simulink model "simIdeal"  (R2023b)
settings: Solver=VariableStepAuto  StartTime=0.0  StopTime=tf  MaxStep=1e-5  RelTol=1e-3
undefined symbols (not defined in the file): ke, p, stepTime, tPWM, Vmax, voltage
libraries: simulink x2
settings Model: Creator=miqui  LastModifiedBy=miqui

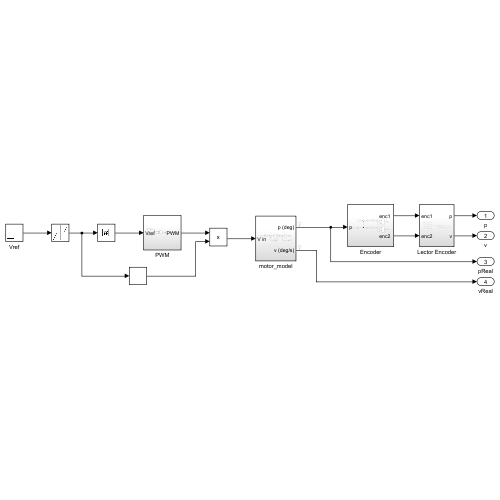
[thumbnail: Simulink's stored preview of the top-level diagram]
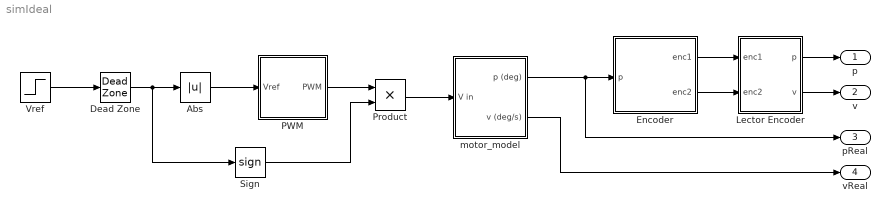
== system simIdeal ==
  Abs : Abs  SaturateOnIntegerOverflow=off
  Dead Zone : DeadZone
  Encoder : Subsystem
  Lector Encoder : Subsystem
  PWM : Subsystem
  Product : Product
  Sign : Signum
  Vref : Step  Time=stepTime  After=voltage  SampleTime=0
  motor_model : Subsystem
  p : Outport
  v : Outport  Port=2
  pReal : Outport  Port=3
  vReal : Outport  Port=4
  wires:
  Dead Zone/1 -> Sign/1, Abs/1
  Abs/1 -> PWM/1(Vref)
  PWM/1(PWM) -> Product/1
  Product/1 -> motor_model/1(V in)
  Sign/1 -> Product/2
  Vref/1 -> Dead Zone/1
  Lector Encoder/2(v) -> v/1
  Lector Encoder/1(p) -> p/1
  motor_model/2(v (deg/s)) -> vReal/1
  motor_model/1(p (deg)) -> Encoder/1(p), pReal/1
  Encoder/1("enc1 ") -> Lector Encoder/1(enc1)
  Encoder/2("enc2 ") -> Lector Encoder/2(enc2)

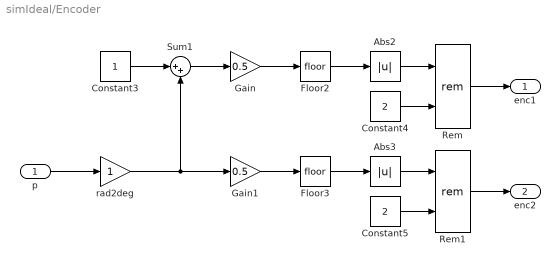
== system simIdeal/Encoder ==
  p : Inport
  Abs2 : Abs  SaturateOnIntegerOverflow=off
  Abs3 : Abs  SaturateOnIntegerOverflow=off
  Constant3 : Constant
  Constant4 : Constant  Value=2
  Constant5 : Constant  Value=2
  Floor2 : Rounding
  Floor3 : Rounding
  Gain : Gain  Gain=0.5
  Gain1 : Gain  Gain=0.5
  Rem : Math  Operator=rem
  Rem1 : Math  Operator=rem
  Sum1 : Sum  Inputs=|++
  rad2deg : Gain
  "enc1 " : Outport  SampleTime=0.0001
  "enc2 " : Outport  Port=2  SampleTime=0.0001
  wires:
  Constant4/1 -> Rem/2
  Constant3/1 -> Sum1/1
  p/1 -> rad2deg/1
  Rem1/1 -> "enc2 "/1
  Gain/1 -> Floor2/1
  Abs3/1 -> Rem1/1
  rad2deg/1 -> Gain1/1, Sum1/2
  Sum1/1 -> Gain/1
  Gain1/1 -> Floor3/1
  Floor3/1 -> Abs3/1
  Floor2/1 -> Abs2/1
  Constant5/1 -> Rem1/2
  Rem/1 -> "enc1 "/1
  Abs2/1 -> Rem/1

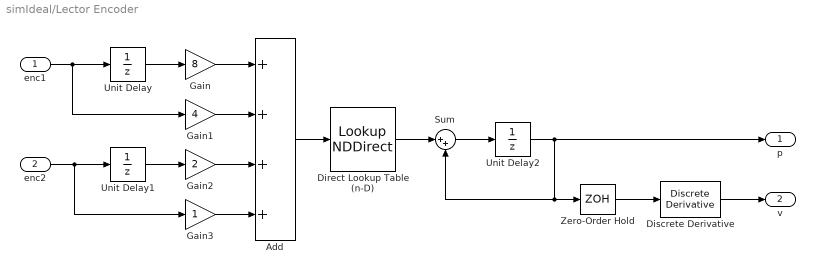
== system simIdeal/Lector Encoder ==
  enc1 : Inport
  enc2 : Inport  Port=2
  Add : Sum  Inputs=++++  OutDataTypeStr=double
  Direct Lookup Table (n-D) : LookupNDDirect  NumberOfTableDimensions=1  Table=[0,-1,1,0,1,0,0,-1,-1,0,0,1,0,1,-1,0]
  Discrete Derivative : simulink/Discrete/Discrete Derivative  gainval=1.0  ICPrevScaledInput=0.0  OutMin=[]  OutMax=[]  OutDataType=fixdt(1, 16)  OutScaling=2^-10  DoSatur=off
  Gain : Gain  Gain=8
  Gain1 : Gain  Gain=4
  Gain2 : Gain  Gain=2
  Gain3 : Gain
  Sum : Sum  Inputs=|++
  Unit Delay : UnitDelay  SampleTime=-1  HasFrameUpgradeWarning=on
  Unit Delay1 : UnitDelay  SampleTime=-1  HasFrameUpgradeWarning=on
  Unit Delay2 : UnitDelay  SampleTime=-1  HasFrameUpgradeWarning=on
  Zero-Order Hold : ZeroOrderHold  SampleTime=0.01
  p : Outport
  v : Outport  Port=2
  wires:
  enc1/1 -> Unit Delay/1, Gain1/1
  enc2/1 -> Unit Delay1/1, Gain3/1
  Unit Delay/1 -> Gain/1
  Unit Delay1/1 -> Gain2/1
  Gain/1 -> Add/1
  Gain1/1 -> Add/2
  Gain2/1 -> Add/3
  Gain3/1 -> Add/4
  Add/1 -> Direct Lookup Table (n-D)/1
  Direct Lookup Table (n-D)/1 -> Sum/1
  Sum/1 -> Unit Delay2/1
  Unit Delay2/1 -> Zero-Order Hold/1, Sum/2, p/1
  Zero-Order Hold/1 -> Discrete Derivative/1
  Discrete Derivative/1 -> v/1

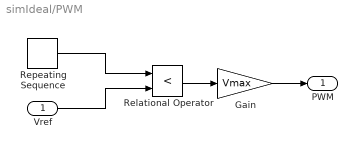
== system simIdeal/PWM ==
  Vref : Inport
  Gain : Gain  Gain=Vmax
  Relational Operator : RelationalOperator  Operator=<  OutDataTypeStr=boolean  RndMeth=Simplest  InputSameDT=off
  Repeating Sequence : simulink/Sources/Repeating Sequence  rep_seq_t=linspace(0,tPWM,100)  rep_seq_y=linspace(0,Vmax,100)
  PWM : Outport
  wires:
  Relational Operator/1 -> Gain/1
  Gain/1 -> PWM/1
  Vref/1 -> Relational Operator/2
  Repeating Sequence/1 -> Relational Operator/1

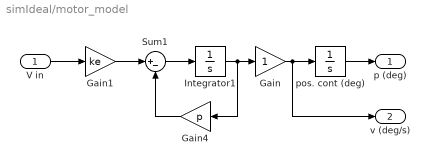
== system simIdeal/motor_model ==
  V in : Inport
  Gain : Gain
  Gain1 : Gain  Gain=ke
  Gain4 : Gain  Gain=p
  Integrator1 : Integrator
  Sum1 : Sum  Inputs=|+-
  pos. cont (deg) : Integrator
  p (deg) : Outport
  v (deg/s) : Outport  Port=2
  wires:
  Sum1/1 -> Integrator1/1
  Gain4/1 -> Sum1/2
  Integrator1/1 -> Gain/1, Gain4/1
  Gain1/1 -> Sum1/1
  Gain/1 -> pos. cont (deg)/1, v (deg/s)/1
  pos. cont (deg)/1 -> p (deg)/1
  V in/1 -> Gain1/1
